simulink model "backstepping2"  (R2021b)
settings: Solver=VariableStepAuto  StartTime=0.0  StopTime=60  RelTol=1e-3
libraries: simulink x1
settings Model: Creator=84232  LastModifiedBy=84232

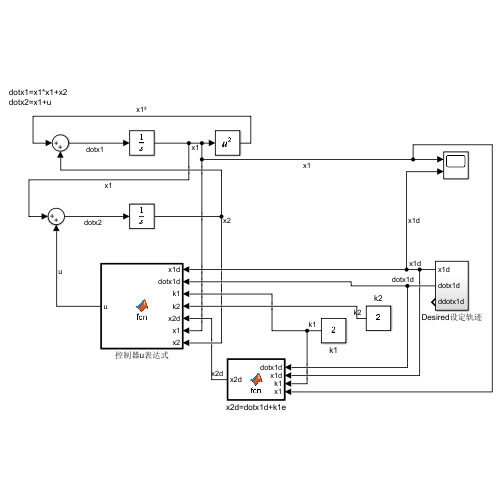
[thumbnail: Simulink's stored preview of the top-level diagram]
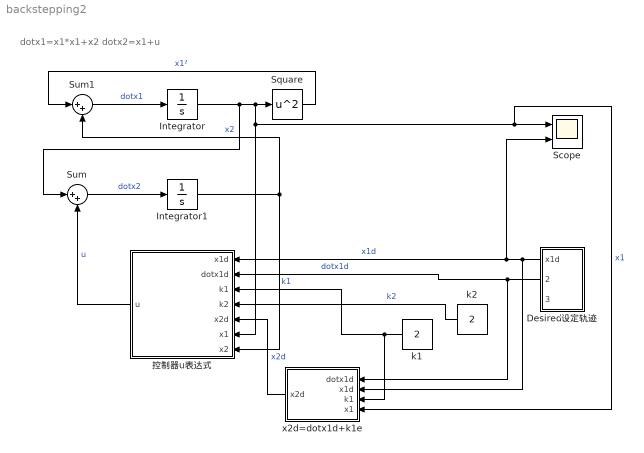
== system backstepping2 ==
  note: dotx1=x1*x1+x2
      | dotx2=x1+u
  Desired设定轨迹 : Subsystem
  Integrator : Integrator
  Integrator1 : Integrator
  Scope : Scope  NumInputPorts=2
  Square : Math  Operator=square  SaturateOnIntegerOverflow=on
  Sum : Sum  Inputs=|++
  Sum1 : Sum  Inputs=|++
  k1 : Constant  Value=2
  k2 : Constant  Value=2
  x2d=dotx1d+k1e : MATLAB Function  TreatAsAtomicUnit=on
  控制器u表达式 : MATLAB Function  TreatAsAtomicUnit=on
  wires:
  Integrator/1 -> Sum/1, x2d=dotx1d+k1e/4(x1), Scope/1, 控制器u表达式/6(x1), Square/1  "x1"
  Sum1/1 -> Integrator/1  "dotx1"
  Sum/1 -> Integrator1/1  "dotx2"
  Square/1 -> Sum1/1  "x1²"
  控制器u表达式/1(u) -> Sum/2  "u"
  Integrator1/1 -> 控制器u表达式/7(x2), Sum1/2  "x2"
  Desired设定轨迹/1(x1d) -> x2d=dotx1d+k1e/2(x1d), Scope/2, 控制器u表达式/1(x1d)  "x1d"
  Desired设定轨迹/2(dotx1d) -> x2d=dotx1d+k1e/1(dotx1d), 控制器u表达式/2(dotx1d)  "dotx1d"
  k2/1 -> 控制器u表达式/4(k2)  "k2"
  k1/1 -> x2d=dotx1d+k1e/3(k1), 控制器u表达式/3(k1)  "k1"
  x2d=dotx1d+k1e/1(x2d) -> 控制器u表达式/5(x2d)  "x2d"

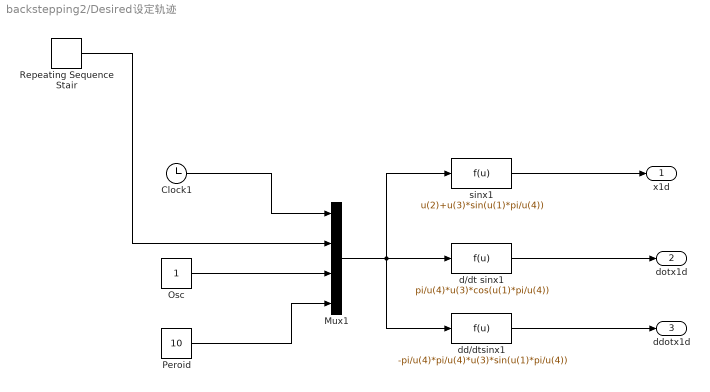
== system backstepping2/Desired设定轨迹 ==
  Clock1 : Clock
      settings: Decimation=100
  Mux1 : Mux
  Osc : Constant
  Peroid : Constant  Value=10
  Repeating Sequence Stair : simulink/Sources/Repeating Sequence Stair  OutValues=[1].'  tsamp=10  OutMin=[]  OutMax=[]  OutDataTypeStr=double  OutputDataTypeScalingMode=double  OutDataType=fixdt(0,8)  ConRadixGroup=Best Precision: Vector-wise  OutScaling=2^-12
  d/dt sinx1 : Fcn  Expr=pi/u(4)*u(3)*cos(u(1)*pi/u(4))
  dd/dtsinx1 : Fcn  Expr=-pi/u(4)*pi/u(4)*u(3)*sin(u(1)*pi/u(4))
  sinx1 : Fcn  Expr=u(2)+u(3)*sin(u(1)*pi/u(4))
  x1d : Outport
  dotx1d : Outport  Port=2
  ddotx1d : Outport  Port=3
  wires:
  Repeating Sequence Stair/1 -> Mux1/2
  Clock1/1 -> Mux1/1
  Mux1/1 -> sinx1/1, dd/dtsinx1/1, d/dt sinx1/1
  Osc/1 -> Mux1/3
  Peroid/1 -> Mux1/4
  d/dt sinx1/1 -> dotx1d/1
  dd/dtsinx1/1 -> ddotx1d/1
  sinx1/1 -> x1d/1

== matlab function backstepping2/控制器u表达式 ==
  data: u output; x1d input; dotx1d input; k1 input; k2 input; x2d input; x1 input; x2 input
function u = fcn(x1d,dotx1d,k1,k2,x2d,x1,x2)

t1=x1d-x1
t2=k1*(x1d-x1)
t3=dotx1d
t4=2*x1*(x1*x1+x2)
t5=x1
t6=k2*(x2d-x2)

u=t1+t2+t3-t4-t5+t6

== matlab function backstepping2/x2d=dotx1d+k1e ==
  data: dotx1d input; x1d input; x2d output; k1 input; x1 input
function x2d = fcn(dotx1d,x1d,k1,x1)


x2d=dotx1d-x1*x1+k1*(x1d-x1);
